simulink model "Q1_part2"  (R2022b)
settings: Solver=VariableStepAuto  StartTime=0.0  StopTime=50  RelTol=1e-3
libraries: mpclib x11, simulink x6, slpidlib x4
settings Model: Creator=Alireza  LastModifiedBy=Alireza

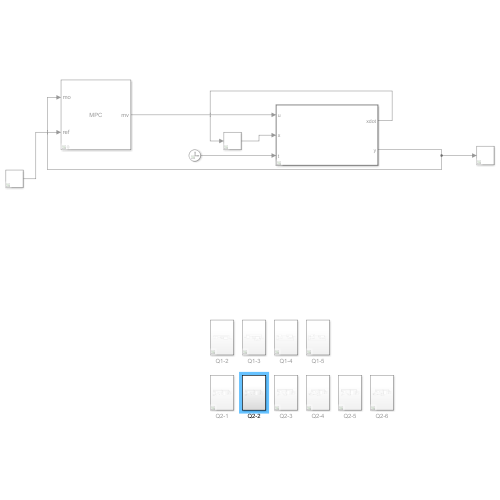
[thumbnail: Simulink's stored preview of the top-level diagram]
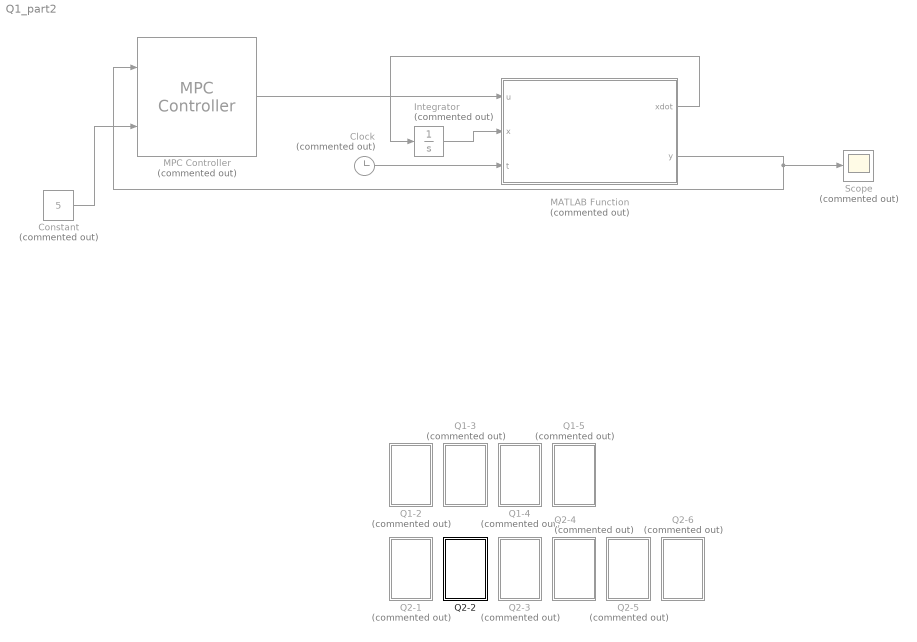
== system Q1_part2 ==
  Clock : Clock  Commented=on
  Constant : Constant  Commented=on  Value=5
  Integrator : Integrator  Commented=on  InitialCondition=[0 0 0 0]
  MATLAB Function : MATLAB Function  Commented=on  TreatAsAtomicUnit=on
  MPC Controller : mpclib/MPC Controller  Commented=on  SCDEnableBlockLinearizationSpecification=on  is_multiple=0  enable_value=0  return_u0=off  updateMPCinCallerWorkspace=on  md_inport=off  mv_inport=off  uref_inport=off  return_cost=off  return_mvseq=off  return_qpstatus=off  return_xseq=off  return_state=off  return_ovseq=off  state_inport=off  umin_inport=off  umax_inport=off  ymin_inport=off  ymax_inport=off  cc_inport=off  ywt_inport=off  uwt_inport=off  duwt_inport=off  rhoeps_inport=off  pm_inport=off  MaximumP=10  HorizonChoice=FixedHorizon  n_ts=0.01  n_p=100  n_mv=1  n_md=1  n_ud=0  n_mo=1  n_uo=0  BlockDataType=double  SampleTimeInherited=off  switch_inport=off
  Q1-2 : Subsystem  Commented=on
  Q1-3 : Subsystem  Commented=on
  Q1-4 : Subsystem  Commented=on
  Q1-5 : Subsystem  Commented=on
  Q2-1 : Subsystem  Commented=on
  Q2-2 : Subsystem
  Q2-3 : Subsystem  Commented=on
  Q2-4 : Subsystem  Commented=on
  Q2-5 : Subsystem  Commented=on
  Q2-6 : Subsystem  Commented=on
  Scope : Scope  Commented=on
  wires:
  Clock/1 -> MATLAB Function/3(t)
  Integrator/1 -> MATLAB Function/2(x)
  MATLAB Function/1(xdot) -> Integrator/1
  MATLAB Function/2(y) -> Scope/1, MPC Controller/1
  Constant/1 -> MPC Controller/2
  MPC Controller/1 -> MATLAB Function/1(u)

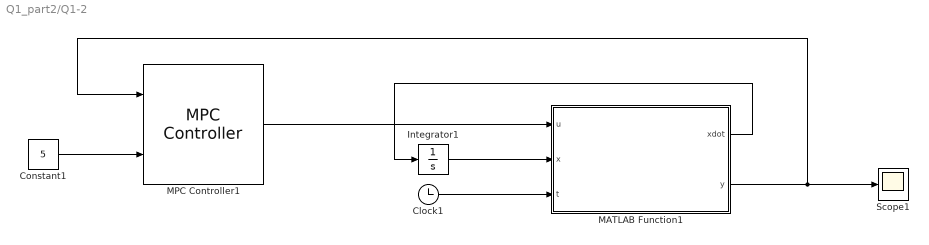
== system Q1_part2/Q1-2 ==
  Clock1 : Clock
  Constant1 : Constant  Value=5
  Integrator1 : Integrator  InitialCondition=[0 0 0 0]
  MATLAB Function1 : MATLAB Function  TreatAsAtomicUnit=on
  MPC Controller1 : mpclib/MPC Controller  SCDEnableBlockLinearizationSpecification=on  mpcobj=mpc1  is_multiple=0  enable_value=0  return_u0=off  updateMPCinCallerWorkspace=on  md_inport=off  mv_inport=off  uref_inport=off  return_cost=off  return_mvseq=off  return_qpstatus=off  return_xseq=off  return_state=off  return_ovseq=off  state_inport=off  umin_inport=off  umax_inport=off  ymin_inport=off  ymax_inport=off  cc_inport=off  ywt_inport=off  uwt_inport=off  duwt_inport=off  rhoeps_inport=off  pm_inport=off  MaximumP=10  HorizonChoice=FixedHorizon  n_ts=0.01  n_p=200  n_mv=1  n_md=0  n_ud=0  n_mo=1  n_uo=0  BlockDataType=double  SampleTimeInherited=off  switch_inport=off
  Scope1 : Scope
  wires:
  Clock1/1 -> MATLAB Function1/3(t)
  MATLAB Function1/2(y) -> MPC Controller1/1, Scope1/1
  Constant1/1 -> MPC Controller1/2
  Integrator1/1 -> MATLAB Function1/2(x)
  MPC Controller1/1 -> MATLAB Function1/1(u)
  MATLAB Function1/1(xdot) -> Integrator1/1

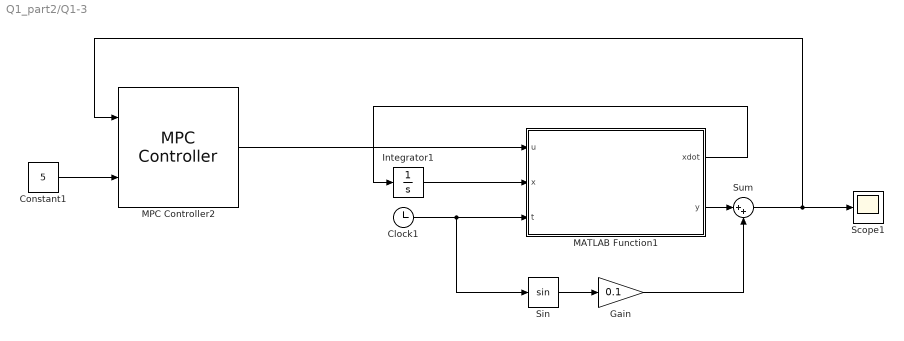
== system Q1_part2/Q1-3 ==
  Clock1 : Clock
  Constant1 : Constant  Value=5
  Gain : Gain  Gain=0.1
  Integrator1 : Integrator  InitialCondition=[0 0 0 0]
  MATLAB Function1 : MATLAB Function  TreatAsAtomicUnit=on
  MPC Controller2 : mpclib/MPC Controller  SCDEnableBlockLinearizationSpecification=on  mpcobj=mpc1  is_multiple=0  enable_value=0  return_u0=off  updateMPCinCallerWorkspace=on  md_inport=off  mv_inport=off  uref_inport=off  return_cost=off  return_mvseq=off  return_qpstatus=off  return_xseq=off  return_state=off  return_ovseq=off  state_inport=off  umin_inport=off  umax_inport=off  ymin_inport=off  ymax_inport=off  cc_inport=off  ywt_inport=off  uwt_inport=off  duwt_inport=off  rhoeps_inport=off  pm_inport=off  MaximumP=10  HorizonChoice=FixedHorizon  n_ts=0.01  n_p=200  n_mv=1  n_md=0  n_ud=0  n_mo=1  n_uo=0  BlockDataType=double  SampleTimeInherited=off  switch_inport=off
  Scope1 : Scope
  Sin : Trigonometry
  Sum : Sum  Inputs=|++
  wires:
  Clock1/1 -> Sin/1, MATLAB Function1/3(t)
  Constant1/1 -> MPC Controller2/2
  Integrator1/1 -> MATLAB Function1/2(x)
  MPC Controller2/1 -> MATLAB Function1/1(u)
  MATLAB Function1/1(xdot) -> Integrator1/1
  Sin/1 -> Gain/1
  Gain/1 -> Sum/2
  MATLAB Function1/2(y) -> Sum/1
  Sum/1 -> MPC Controller2/1, Scope1/1

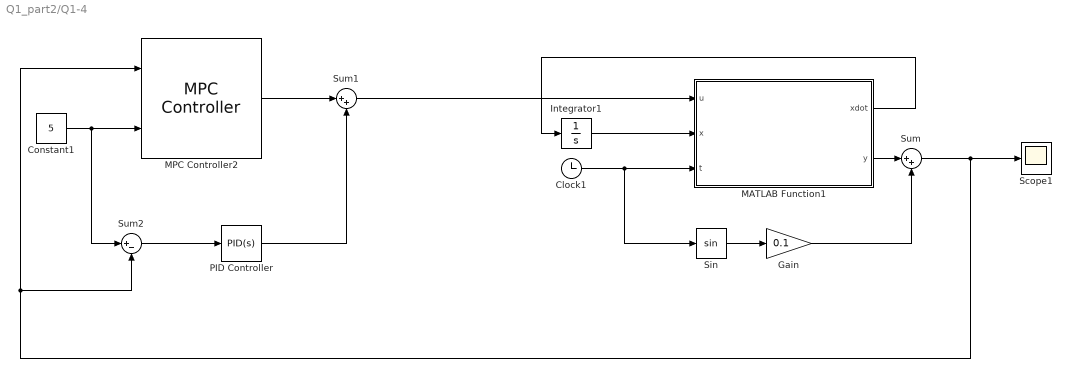
== system Q1_part2/Q1-4 ==
  Clock1 : Clock
  Constant1 : Constant  Value=5
  Gain : Gain  Gain=0.1
  Integrator1 : Integrator  InitialCondition=[0 0 0 0]
  MATLAB Function1 : MATLAB Function  TreatAsAtomicUnit=on
  MPC Controller2 : mpclib/MPC Controller  SCDEnableBlockLinearizationSpecification=on  mpcobj=mpc1  is_multiple=0  enable_value=0  return_u0=off  updateMPCinCallerWorkspace=on  md_inport=off  mv_inport=off  uref_inport=off  return_cost=off  return_mvseq=off  return_qpstatus=off  return_xseq=off  return_state=off  return_ovseq=off  state_inport=off  umin_inport=off  umax_inport=off  ymin_inport=off  ymax_inport=off  cc_inport=off  ywt_inport=off  uwt_inport=off  duwt_inport=off  rhoeps_inport=off  pm_inport=off  MaximumP=10  HorizonChoice=FixedHorizon  n_ts=0.01  n_p=200  n_mv=1  n_md=0  n_ud=0  n_mo=1  n_uo=0  BlockDataType=double  SampleTimeInherited=off  switch_inport=off
  PID Controller : slpidlib/PID Controller  Controller=PID  Form=Parallel  TimeDomain=Continuous-time  UseExternalTs=off  SampleTime=-1  IntegratorMethod=Forward Euler  FilterMethod=Forward Euler  ControllerParametersSource=internal  P=14.0581841806132  I=1.12903294333541  UseKiTs=off  D=19.0426786123122  N=1197.69951514709  UseFilter=on  TunerSelectOption=Transfer Function Based (PID Tuner App)  InitialConditionSource=internal  InitialConditionForIntegrator=0  InitialConditionForFilter=0  DifferentiatorICPrevScaledInput=0  ExternalReset=none  TrackingMode=off  Kt=1  LimitOutput=off  SatLimitsSource=internal  UpperSaturationLimit=inf  LowerSaturationLimit=-inf  LinearizeAsGain=on  AntiWindupMode=none  Kb=1  LimitIntegrator=off  UpperIntegratorSaturationLimit=inf  LowerIntegratorSaturationLimit=-inf  POutMin=[]  POutMax=[]  IOutMin=[]  IOutMax=[]  DOutMin=[]  DOutMax=[]  NOutMin=[]  NOutMax=[]  SumOutMin=[]  SumOutMax=[]  SaturationOutMin=[]  SaturationOutMax=[]  PParamMin=[]  PParamMax=[]  IParamMin=[]  IParamMax=[]  DParamMin=[]  DParamMax=[]  NParamMin=[]  NParamMax=[]  KbParamMin=[]  KbParamMax=[]  KtParamMin=[]  KtParamMax=[]  KbOutMin=[]  KbOutMax=[]  KtOutMin=[]  KtOutMax=[]  IntegratorOutMin=[]  IntegratorOutMax=[]  FilterOutMin=[]  FilterOutMax=[]  SumI1OutMin=[]  SumI1OutMax=[]  SumI2OutMin=[]  SumI2OutMax=[]  SumI3OutMin=[]  SumI3OutMax=[]  SumI4OutMin=[]  SumI4OutMax=[]  SumDOutMin=[]  SumDOutMax=[]  DifferentiatorOutMin=[]  DifferentiatorOutMax=[]  FilterDiffOutCoefMin=[]  FilterDiffOutCoefMax=[]  ReciprocalOutMin=[]  ReciprocalOutMax=[]  SumDenOutMin=[]  SumDenOutMax=[]  SumNumOutMin=[]  SumNumOutMax=[]  DivideOutMin=[]  DivideOutMax=[]  UdiffTsProdOutMin=[]  UdiffTsProdOutMax=[]  NTsProdOutMin=[]  NTsProdOutMax=[]  UintegralTsProdOutMin=[]  UintegralTsProdOutMax=[]  UngainTsProdOutMin=[]  UngainTsProdOutMax=[]  ClampingZeroOutDataTypeStr=Inherit: Inherit via back propagation  ClampingZeroOutMin=[]  ClampingZeroOutMax=[]  FilterDenConstantOutDataTypeStr=Inherit: Inherit via back propagation  FilterDenConstantOutMin=[]  FilterDenConstantOutMax=[]  PCopyOutDataTypeStr=Inherit: Inherit via back propagation  PCopyOutMin=[]  PCopyOutMax=[]  NCopyOutDataTypeStr=Inherit: Inherit via back propagation  NCopyOutMin=[]  NCopyOutMax=[]  IntegratorContinuousStateAttributes=''  IntegratorStateMustResolveToSignalObject=off  IntegratorRTWStateStorageClass=Auto  FilterContinuousStateAttributes=''  FilterStateMustResolveToSignalObject=off  FilterRTWStateStorageClass=Auto  ParallelPVariant=InternalParameters  IdealPVariant=Disabled  IVariant=InternalParameters  DVariant=InternalParameters  IntegratorVariant=Continuous  SatVariant=Disabled  AWVariant=Passthrough  PCopyVariant=Disabled  TRVariant=Disabled  FdbkBlocksVariant=Forward  IdealPFdbkVariant=Disabled  SatFdbkVariant=Disabled  DerivativeFilterVariant=ContFilter  NVariant=InternalParameters  NCopyVariant=Disabled  FilterICVariant=InternalICsFilter  IntegratorICVariant=InternalICs  ExternalResetVariant=Disabled  TRSumVariant=Passthrough  SumFdbkVariant=Disabled  SumVariant=Sum_PID  TsampFilterVariant=InternalTs  TsampNgainVariant=Passthrough  TsampIntegralVariant=Passthrough  ExternalSaturationOutDataTypeStr=Inherit: Same as second input
  Scope1 : Scope
  Sin : Trigonometry
  Sum : Sum  Inputs=|++
  Sum1 : Sum  Inputs=|++
  Sum2 : Sum  Inputs=|+-
  wires:
  Sum/1 -> Scope1/1, MPC Controller2/1, Sum2/2
  MATLAB Function1/2(y) -> Sum/1
  Gain/1 -> Sum/2
  Sin/1 -> Gain/1
  MATLAB Function1/1(xdot) -> Integrator1/1
  Integrator1/1 -> MATLAB Function1/2(x)
  Constant1/1 -> Sum2/1, MPC Controller2/2
  Clock1/1 -> MATLAB Function1/3(t), Sin/1
  MPC Controller2/1 -> Sum1/1
  PID Controller/1 -> Sum1/2
  Sum1/1 -> MATLAB Function1/1(u)
  Sum2/1 -> PID Controller/1

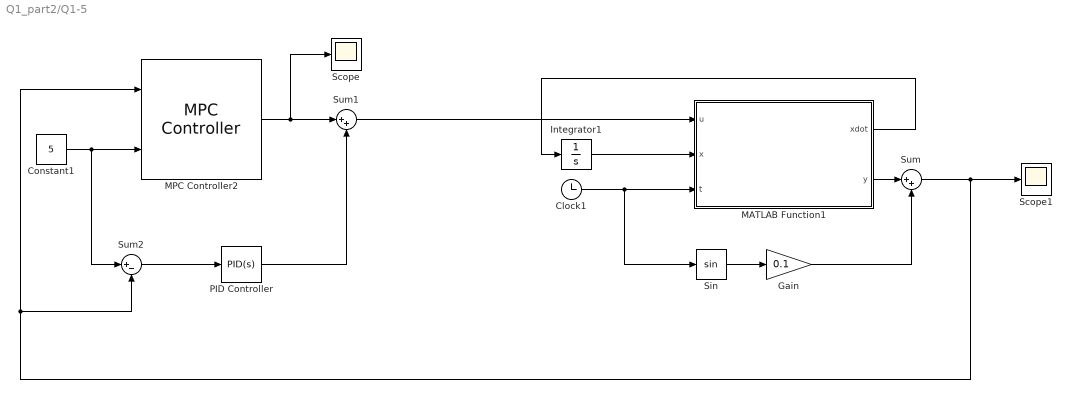
== system Q1_part2/Q1-5 ==
  Clock1 : Clock
  Constant1 : Constant  Value=5
  Gain : Gain  Gain=0.1
  Integrator1 : Integrator  InitialCondition=[0 0 0 0]
  MATLAB Function1 : MATLAB Function  TreatAsAtomicUnit=on
  MPC Controller2 : mpclib/MPC Controller  SCDEnableBlockLinearizationSpecification=on  mpcobj=mpc2  is_multiple=0  enable_value=0  return_u0=off  updateMPCinCallerWorkspace=on  md_inport=off  mv_inport=off  uref_inport=off  return_cost=off  return_mvseq=off  return_qpstatus=off  return_xseq=off  return_state=off  return_ovseq=off  state_inport=off  umin_inport=off  umax_inport=off  ymin_inport=off  ymax_inport=off  cc_inport=off  ywt_inport=off  uwt_inport=off  duwt_inport=off  rhoeps_inport=off  pm_inport=off  MaximumP=10  HorizonChoice=FixedHorizon  n_ts=0.01  n_p=200  n_mv=1  n_md=0  n_ud=0  n_mo=1  n_uo=0  BlockDataType=double  SampleTimeInherited=off  switch_inport=off
  PID Controller : slpidlib/PID Controller  Controller=PID  Form=Parallel  TimeDomain=Continuous-time  UseExternalTs=off  SampleTime=-1  IntegratorMethod=Forward Euler  FilterMethod=Forward Euler  ControllerParametersSource=internal  P=14.0581841806132  I=1.12903294333541  UseKiTs=off  D=19.0426786123122  N=1197.69951514709  UseFilter=on  TunerSelectOption=Transfer Function Based (PID Tuner App)  InitialConditionSource=internal  InitialConditionForIntegrator=0  InitialConditionForFilter=0  DifferentiatorICPrevScaledInput=0  ExternalReset=none  TrackingMode=off  Kt=1  LimitOutput=off  SatLimitsSource=internal  UpperSaturationLimit=inf  LowerSaturationLimit=-inf  LinearizeAsGain=on  AntiWindupMode=none  Kb=1  LimitIntegrator=off  UpperIntegratorSaturationLimit=inf  LowerIntegratorSaturationLimit=-inf  POutMin=[]  POutMax=[]  IOutMin=[]  IOutMax=[]  DOutMin=[]  DOutMax=[]  NOutMin=[]  NOutMax=[]  SumOutMin=[]  SumOutMax=[]  SaturationOutMin=[]  SaturationOutMax=[]  PParamMin=[]  PParamMax=[]  IParamMin=[]  IParamMax=[]  DParamMin=[]  DParamMax=[]  NParamMin=[]  NParamMax=[]  KbParamMin=[]  KbParamMax=[]  KtParamMin=[]  KtParamMax=[]  KbOutMin=[]  KbOutMax=[]  KtOutMin=[]  KtOutMax=[]  IntegratorOutMin=[]  IntegratorOutMax=[]  FilterOutMin=[]  FilterOutMax=[]  SumI1OutMin=[]  SumI1OutMax=[]  SumI2OutMin=[]  SumI2OutMax=[]  SumI3OutMin=[]  SumI3OutMax=[]  SumI4OutMin=[]  SumI4OutMax=[]  SumDOutMin=[]  SumDOutMax=[]  DifferentiatorOutMin=[]  DifferentiatorOutMax=[]  FilterDiffOutCoefMin=[]  FilterDiffOutCoefMax=[]  ReciprocalOutMin=[]  ReciprocalOutMax=[]  SumDenOutMin=[]  SumDenOutMax=[]  SumNumOutMin=[]  SumNumOutMax=[]  DivideOutMin=[]  DivideOutMax=[]  UdiffTsProdOutMin=[]  UdiffTsProdOutMax=[]  NTsProdOutMin=[]  NTsProdOutMax=[]  UintegralTsProdOutMin=[]  UintegralTsProdOutMax=[]  UngainTsProdOutMin=[]  UngainTsProdOutMax=[]  ClampingZeroOutDataTypeStr=Inherit: Inherit via back propagation  ClampingZeroOutMin=[]  ClampingZeroOutMax=[]  FilterDenConstantOutDataTypeStr=Inherit: Inherit via back propagation  FilterDenConstantOutMin=[]  FilterDenConstantOutMax=[]  PCopyOutDataTypeStr=Inherit: Inherit via back propagation  PCopyOutMin=[]  PCopyOutMax=[]  NCopyOutDataTypeStr=Inherit: Inherit via back propagation  NCopyOutMin=[]  NCopyOutMax=[]  IntegratorContinuousStateAttributes=''  IntegratorStateMustResolveToSignalObject=off  IntegratorRTWStateStorageClass=Auto  FilterContinuousStateAttributes=''  FilterStateMustResolveToSignalObject=off  FilterRTWStateStorageClass=Auto  ParallelPVariant=InternalParameters  IdealPVariant=Disabled  IVariant=InternalParameters  DVariant=InternalParameters  IntegratorVariant=Continuous  SatVariant=Disabled  AWVariant=Passthrough  PCopyVariant=Disabled  TRVariant=Disabled  FdbkBlocksVariant=Forward  IdealPFdbkVariant=Disabled  SatFdbkVariant=Disabled  DerivativeFilterVariant=ContFilter  NVariant=InternalParameters  NCopyVariant=Disabled  FilterICVariant=InternalICsFilter  IntegratorICVariant=InternalICs  ExternalResetVariant=Disabled  TRSumVariant=Passthrough  SumFdbkVariant=Disabled  SumVariant=Sum_PID  TsampFilterVariant=InternalTs  TsampNgainVariant=Passthrough  TsampIntegralVariant=Passthrough  ExternalSaturationOutDataTypeStr=Inherit: Same as second input
  Scope : Scope
  Scope1 : Scope
  Sin : Trigonometry
  Sum : Sum  Inputs=|++
  Sum1 : Sum  Inputs=|++
  Sum2 : Sum  Inputs=|+-
  wires:
  Sum2/1 -> PID Controller/1
  Sum1/1 -> MATLAB Function1/1(u)
  PID Controller/1 -> Sum1/2
  MPC Controller2/1 -> Scope/1, Sum1/1
  Clock1/1 -> Sin/1, MATLAB Function1/3(t)
  Constant1/1 -> MPC Controller2/2, Sum2/1
  Integrator1/1 -> MATLAB Function1/2(x)
  MATLAB Function1/1(xdot) -> Integrator1/1
  Sin/1 -> Gain/1
  Gain/1 -> Sum/2
  MATLAB Function1/2(y) -> Sum/1
  Sum/1 -> Sum2/2, MPC Controller2/1, Scope1/1

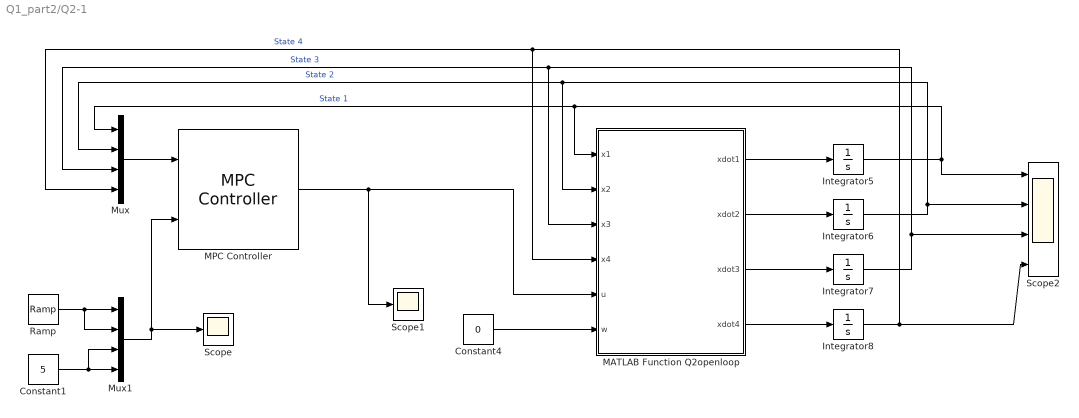
== system Q1_part2/Q2-1 ==
  Constant1 : Constant  Value=5
  Constant4 : Constant  Value=0
  Integrator{5..8} (4 alike) : Integrator
  MATLAB Function Q2openloop : MATLAB Function  TreatAsAtomicUnit=on
  MPC Controller : mpclib/MPC Controller  SCDEnableBlockLinearizationSpecification=on  mpcobj=mpc1  is_multiple=0  enable_value=0  return_u0=off  updateMPCinCallerWorkspace=on  md_inport=off  mv_inport=off  uref_inport=off  return_cost=off  return_mvseq=off  return_qpstatus=off  return_xseq=off  return_state=off  return_ovseq=off  state_inport=off  umin_inport=off  umax_inport=off  ymin_inport=off  ymax_inport=off  cc_inport=off  ywt_inport=off  uwt_inport=off  duwt_inport=off  rhoeps_inport=off  pm_inport=off  MaximumP=10  HorizonChoice=FixedHorizon  n_ts=0.01  n_p=650  n_mv=1  n_md=0  n_ud=0  n_mo=4  n_uo=0  BlockDataType=double  SampleTimeInherited=off  switch_inport=off
  Mux : Mux
  Mux1 : Mux
  Ramp : simulink/Sources/Ramp  slope=1  start=0  InitialOutput=0
  Scope : Scope
  Scope1 : Scope
  Scope2 : Scope  NumInputPorts=4
  wires:
  Mux/1 -> MPC Controller/1
  Ramp/1 -> Mux1/2, Mux1/1
  Constant1/1 -> Mux1/4, Mux1/3
  Mux1/1 -> Scope/1, MPC Controller/2
  Integrator5/1 -> Scope2/1, Mux/1, MATLAB Function Q2openloop/1(x1)  "State 1"
  MATLAB Function Q2openloop/1(xdot1) -> Integrator5/1
  Integrator7/1 -> Scope2/3, MATLAB Function Q2openloop/3(x3), Mux/3  "State 3"
  Integrator6/1 -> Scope2/2, MATLAB Function Q2openloop/2(x2), Mux/2  "State 2"
  MATLAB Function Q2openloop/3(xdot3) -> Integrator7/1
  MATLAB Function Q2openloop/4(xdot4) -> Integrator8/1
  MATLAB Function Q2openloop/2(xdot2) -> Integrator6/1
  Integrator8/1 -> MATLAB Function Q2openloop/4(x4), Mux/4, Scope2/4  "State 4"
  Constant4/1 -> MATLAB Function Q2openloop/6(w)
  MPC Controller/1 -> MATLAB Function Q2openloop/5(u), Scope1/1

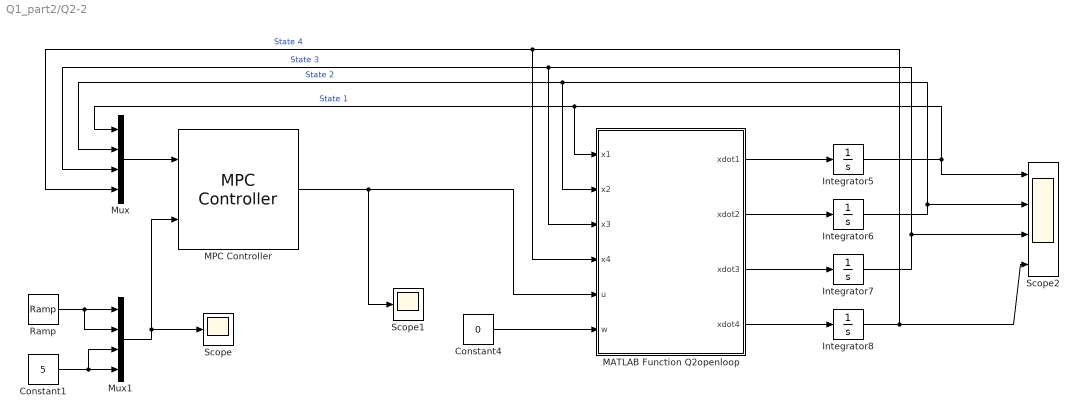
== system Q1_part2/Q2-2 ==
  Constant1 : Constant  Value=5
  Constant4 : Constant  Value=0
  Integrator{5..8} (4 alike) : Integrator
  MATLAB Function Q2openloop : MATLAB Function  TreatAsAtomicUnit=on
  MPC Controller : mpclib/MPC Controller  SCDEnableBlockLinearizationSpecification=on  mpcobj=mpc1  is_multiple=0  enable_value=0  return_u0=off  updateMPCinCallerWorkspace=on  md_inport=off  mv_inport=off  uref_inport=off  return_cost=off  return_mvseq=off  return_qpstatus=off  return_xseq=off  return_state=off  return_ovseq=off  state_inport=off  umin_inport=off  umax_inport=off  ymin_inport=off  ymax_inport=off  cc_inport=off  ywt_inport=off  uwt_inport=off  duwt_inport=off  rhoeps_inport=off  pm_inport=off  MaximumP=10  HorizonChoice=FixedHorizon  n_ts=0.01  n_p=650  n_mv=1  n_md=0  n_ud=0  n_mo=4  n_uo=0  BlockDataType=double  SampleTimeInherited=off  switch_inport=off
  Mux : Mux
  Mux1 : Mux
  Ramp : simulink/Sources/Ramp  slope=1  start=0  InitialOutput=0
  Scope : Scope
  Scope1 : Scope
  Scope2 : Scope  NumInputPorts=4
  wires:
  MPC Controller/1 -> Scope1/1, MATLAB Function Q2openloop/5(u)
  Constant4/1 -> MATLAB Function Q2openloop/6(w)
  Integrator8/1 -> Scope2/4, Mux/4, MATLAB Function Q2openloop/4(x4)  "State 4"
  MATLAB Function Q2openloop/2(xdot2) -> Integrator6/1
  MATLAB Function Q2openloop/4(xdot4) -> Integrator8/1
  MATLAB Function Q2openloop/3(xdot3) -> Integrator7/1
  Integrator6/1 -> Mux/2, MATLAB Function Q2openloop/2(x2), Scope2/2  "State 2"
  Integrator7/1 -> Mux/3, MATLAB Function Q2openloop/3(x3), Scope2/3  "State 3"
  MATLAB Function Q2openloop/1(xdot1) -> Integrator5/1
  Integrator5/1 -> MATLAB Function Q2openloop/1(x1), Mux/1, Scope2/1  "State 1"
  Mux1/1 -> MPC Controller/2, Scope/1
  Constant1/1 -> Mux1/3, Mux1/4
  Ramp/1 -> Mux1/1, Mux1/2
  Mux/1 -> MPC Controller/1

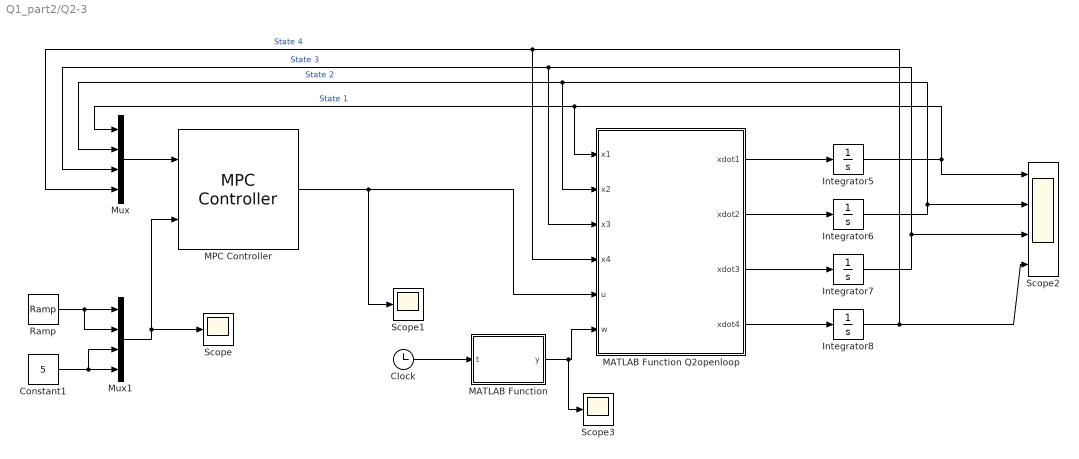
== system Q1_part2/Q2-3 ==
  Clock : Clock
  Constant1 : Constant  Value=5
  Integrator{5..8} (4 alike) : Integrator
  MATLAB Function : MATLAB Function  TreatAsAtomicUnit=on
  MATLAB Function Q2openloop : MATLAB Function  TreatAsAtomicUnit=on
  MPC Controller : mpclib/MPC Controller  SCDEnableBlockLinearizationSpecification=on  mpcobj=mpc1  is_multiple=0  enable_value=0  return_u0=off  updateMPCinCallerWorkspace=on  md_inport=off  mv_inport=off  uref_inport=off  return_cost=off  return_mvseq=off  return_qpstatus=off  return_xseq=off  return_state=off  return_ovseq=off  state_inport=off  umin_inport=off  umax_inport=off  ymin_inport=off  ymax_inport=off  cc_inport=off  ywt_inport=off  uwt_inport=off  duwt_inport=off  rhoeps_inport=off  pm_inport=off  MaximumP=10  HorizonChoice=FixedHorizon  n_ts=0.01  n_p=650  n_mv=1  n_md=0  n_ud=0  n_mo=4  n_uo=0  BlockDataType=double  SampleTimeInherited=off  switch_inport=off
  Mux : Mux
  Mux1 : Mux
  Ramp : simulink/Sources/Ramp  slope=1  start=0  InitialOutput=0
  Scope : Scope
  Scope1 : Scope
  Scope2 : Scope  NumInputPorts=4
  Scope3 : Scope
  wires:
  Mux/1 -> MPC Controller/1
  Ramp/1 -> Mux1/2, Mux1/1
  Constant1/1 -> Mux1/4, Mux1/3
  Mux1/1 -> Scope/1, MPC Controller/2
  Integrator5/1 -> Scope2/1, Mux/1, MATLAB Function Q2openloop/1(x1)  "State 1"
  MATLAB Function Q2openloop/1(xdot1) -> Integrator5/1
  Integrator7/1 -> Scope2/3, MATLAB Function Q2openloop/3(x3), Mux/3  "State 3"
  Integrator6/1 -> Scope2/2, MATLAB Function Q2openloop/2(x2), Mux/2  "State 2"
  MATLAB Function Q2openloop/3(xdot3) -> Integrator7/1
  MATLAB Function Q2openloop/4(xdot4) -> Integrator8/1
  MATLAB Function Q2openloop/2(xdot2) -> Integrator6/1
  Integrator8/1 -> MATLAB Function Q2openloop/4(x4), Mux/4, Scope2/4  "State 4"
  MPC Controller/1 -> MATLAB Function Q2openloop/5(u), Scope1/1
  MATLAB Function/1(y) -> Scope3/1, MATLAB Function Q2openloop/6(w)
  Clock/1 -> MATLAB Function/1(t)

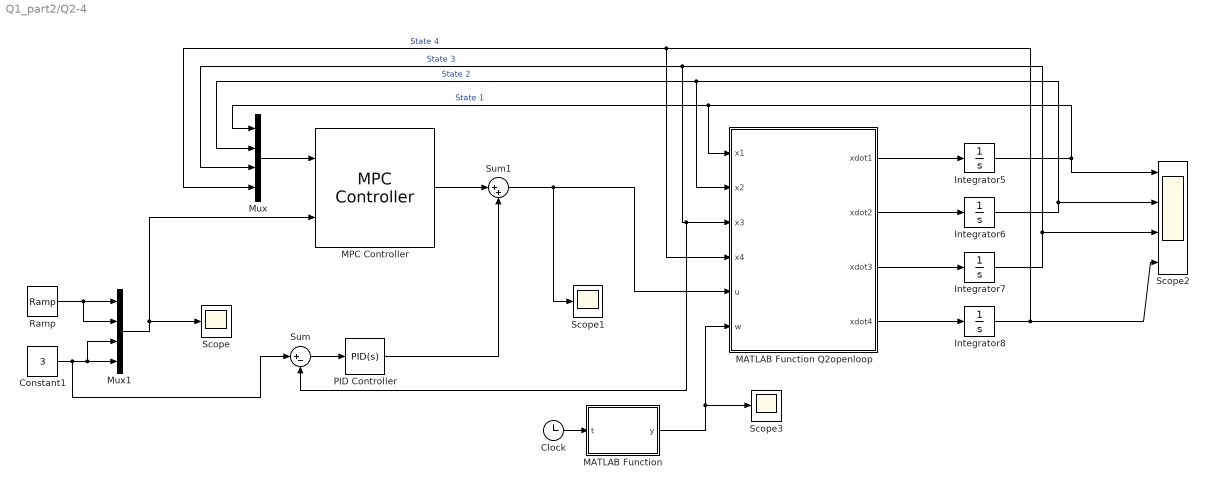
== system Q1_part2/Q2-4 ==
  Clock : Clock
  Constant1 : Constant  Value=3
  Integrator{5..8} (4 alike) : Integrator
  MATLAB Function : MATLAB Function  TreatAsAtomicUnit=on
  MATLAB Function Q2openloop : MATLAB Function  TreatAsAtomicUnit=on
  MPC Controller : mpclib/MPC Controller  SCDEnableBlockLinearizationSpecification=on  mpcobj=mpc1  is_multiple=0  enable_value=0  return_u0=off  updateMPCinCallerWorkspace=on  md_inport=off  mv_inport=off  uref_inport=off  return_cost=off  return_mvseq=off  return_qpstatus=off  return_xseq=off  return_state=off  return_ovseq=off  state_inport=off  umin_inport=off  umax_inport=off  ymin_inport=off  ymax_inport=off  cc_inport=off  ywt_inport=off  uwt_inport=off  duwt_inport=off  rhoeps_inport=off  pm_inport=off  MaximumP=10  HorizonChoice=FixedHorizon  n_ts=0.01  n_p=650  n_mv=1  n_md=0  n_ud=0  n_mo=4  n_uo=0  BlockDataType=double  SampleTimeInherited=off  switch_inport=off
  Mux : Mux
  Mux1 : Mux
  PID Controller : slpidlib/PID Controller  Controller=PID  Form=Parallel  TimeDomain=Continuous-time  UseExternalTs=off  SampleTime=-1  IntegratorMethod=Forward Euler  FilterMethod=Forward Euler  ControllerParametersSource=internal  P=200  I=10  UseKiTs=off  D=100  N=100  UseFilter=on  TunerSelectOption=Transfer Function Based (PID Tuner App)  InitialConditionSource=internal  InitialConditionForIntegrator=0  InitialConditionForFilter=0  DifferentiatorICPrevScaledInput=0  ExternalReset=none  TrackingMode=off  Kt=1  LimitOutput=off  SatLimitsSource=internal  UpperSaturationLimit=inf  LowerSaturationLimit=-inf  LinearizeAsGain=on  AntiWindupMode=none  Kb=1  LimitIntegrator=off  UpperIntegratorSaturationLimit=inf  LowerIntegratorSaturationLimit=-inf  POutMin=[]  POutMax=[]  IOutMin=[]  IOutMax=[]  DOutMin=[]  DOutMax=[]  NOutMin=[]  NOutMax=[]  SumOutMin=[]  SumOutMax=[]  SaturationOutMin=[]  SaturationOutMax=[]  PParamMin=[]  PParamMax=[]  IParamMin=[]  IParamMax=[]  DParamMin=[]  DParamMax=[]  NParamMin=[]  NParamMax=[]  KbParamMin=[]  KbParamMax=[]  KtParamMin=[]  KtParamMax=[]  KbOutMin=[]  KbOutMax=[]  KtOutMin=[]  KtOutMax=[]  IntegratorOutMin=[]  IntegratorOutMax=[]  FilterOutMin=[]  FilterOutMax=[]  SumI1OutMin=[]  SumI1OutMax=[]  SumI2OutMin=[]  SumI2OutMax=[]  SumI3OutMin=[]  SumI3OutMax=[]  SumI4OutMin=[]  SumI4OutMax=[]  SumDOutMin=[]  SumDOutMax=[]  DifferentiatorOutMin=[]  DifferentiatorOutMax=[]  FilterDiffOutCoefMin=[]  FilterDiffOutCoefMax=[]  ReciprocalOutMin=[]  ReciprocalOutMax=[]  SumDenOutMin=[]  SumDenOutMax=[]  SumNumOutMin=[]  SumNumOutMax=[]  DivideOutMin=[]  DivideOutMax=[]  UdiffTsProdOutMin=[]  UdiffTsProdOutMax=[]  NTsProdOutMin=[]  NTsProdOutMax=[]  UintegralTsProdOutMin=[]  UintegralTsProdOutMax=[]  UngainTsProdOutMin=[]  UngainTsProdOutMax=[]  ClampingZeroOutDataTypeStr=Inherit: Inherit via back propagation  ClampingZeroOutMin=[]  ClampingZeroOutMax=[]  FilterDenConstantOutDataTypeStr=Inherit: Inherit via back propagation  FilterDenConstantOutMin=[]  FilterDenConstantOutMax=[]  PCopyOutDataTypeStr=Inherit: Inherit via back propagation  PCopyOutMin=[]  PCopyOutMax=[]  NCopyOutDataTypeStr=Inherit: Inherit via back propagation  NCopyOutMin=[]  NCopyOutMax=[]  IntegratorContinuousStateAttributes=''  IntegratorStateMustResolveToSignalObject=off  IntegratorRTWStateStorageClass=Auto  FilterContinuousStateAttributes=''  FilterStateMustResolveToSignalObject=off  FilterRTWStateStorageClass=Auto  ParallelPVariant=InternalParameters  IdealPVariant=Disabled  IVariant=InternalParameters  DVariant=InternalParameters  IntegratorVariant=Continuous  SatVariant=Disabled  AWVariant=Passthrough  PCopyVariant=Disabled  TRVariant=Disabled  FdbkBlocksVariant=Forward  IdealPFdbkVariant=Disabled  SatFdbkVariant=Disabled  DerivativeFilterVariant=ContFilter  NVariant=InternalParameters  NCopyVariant=Disabled  FilterICVariant=InternalICsFilter  IntegratorICVariant=InternalICs  ExternalResetVariant=Disabled  TRSumVariant=Passthrough  SumFdbkVariant=Disabled  SumVariant=Sum_PID  TsampFilterVariant=InternalTs  TsampNgainVariant=Passthrough  TsampIntegralVariant=Passthrough  ExternalSaturationOutDataTypeStr=Inherit: Same as second input
  Ramp : simulink/Sources/Ramp  slope=1  start=0  InitialOutput=0
  Scope : Scope
  Scope1 : Scope
  Scope2 : Scope  NumInputPorts=4
  Scope3 : Scope
  Sum : Sum  Inputs=|+-
  Sum1 : Sum  Inputs=|++
  wires:
  Clock/1 -> MATLAB Function/1(t)
  MATLAB Function/1(y) -> Scope3/1, MATLAB Function Q2openloop/6(w)
  Integrator8/1 -> Scope2/4, Mux/4, MATLAB Function Q2openloop/4(x4)  "State 4"
  MATLAB Function Q2openloop/2(xdot2) -> Integrator6/1
  MATLAB Function Q2openloop/4(xdot4) -> Integrator8/1
  MATLAB Function Q2openloop/3(xdot3) -> Integrator7/1
  Integrator6/1 -> Mux/2, MATLAB Function Q2openloop/2(x2), Scope2/2  "State 2"
  Integrator7/1 -> Mux/3, MATLAB Function Q2openloop/3(x3), Sum/2, Scope2/3  "State 3"
  MATLAB Function Q2openloop/1(xdot1) -> Integrator5/1
  Integrator5/1 -> MATLAB Function Q2openloop/1(x1), Mux/1, Scope2/1  "State 1"
  Mux1/1 -> MPC Controller/2, Scope/1
  Constant1/1 -> Sum/1, Mux1/3, Mux1/4
  Ramp/1 -> Mux1/1, Mux1/2
  Mux/1 -> MPC Controller/1
  Sum/1 -> PID Controller/1
  MPC Controller/1 -> Sum1/1
  Sum1/1 -> Scope1/1, MATLAB Function Q2openloop/5(u)
  PID Controller/1 -> Sum1/2

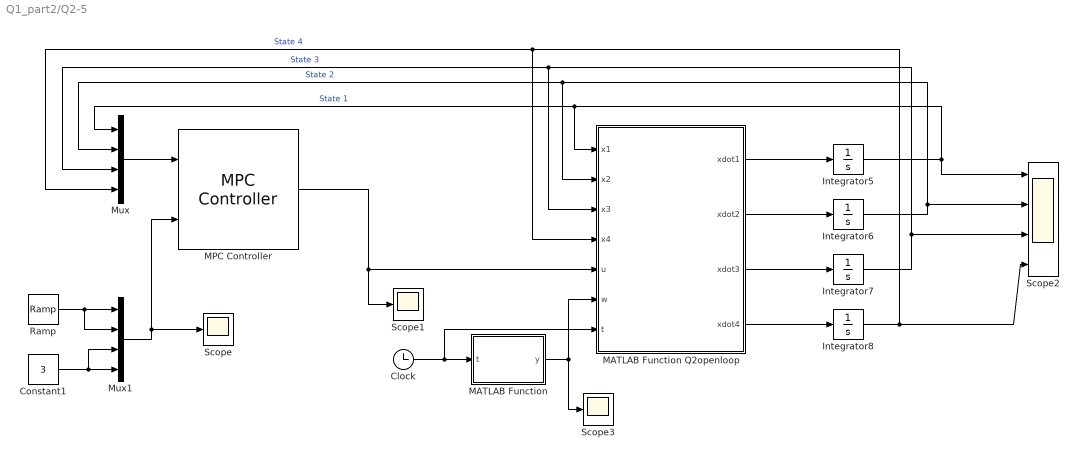
== system Q1_part2/Q2-5 ==
  Clock : Clock
  Constant1 : Constant  Value=3
  Integrator{5..8} (4 alike) : Integrator
  MATLAB Function : MATLAB Function  TreatAsAtomicUnit=on
  MATLAB Function Q2openloop : MATLAB Function  TreatAsAtomicUnit=on
  MPC Controller : mpclib/MPC Controller  SCDEnableBlockLinearizationSpecification=on  mpcobj=mpc1  is_multiple=0  enable_value=0  return_u0=off  updateMPCinCallerWorkspace=on  md_inport=off  mv_inport=off  uref_inport=off  return_cost=off  return_mvseq=off  return_qpstatus=off  return_xseq=off  return_state=off  return_ovseq=off  state_inport=off  umin_inport=off  umax_inport=off  ymin_inport=off  ymax_inport=off  cc_inport=off  ywt_inport=off  uwt_inport=off  duwt_inport=off  rhoeps_inport=off  pm_inport=off  MaximumP=10  HorizonChoice=FixedHorizon  n_ts=0.01  n_p=650  n_mv=1  n_md=0  n_ud=0  n_mo=4  n_uo=0  BlockDataType=double  SampleTimeInherited=off  switch_inport=off
  Mux : Mux
  Mux1 : Mux
  Ramp : simulink/Sources/Ramp  slope=1  start=0  InitialOutput=0
  Scope : Scope
  Scope1 : Scope
  Scope2 : Scope  NumInputPorts=4
  Scope3 : Scope
  wires:
  Clock/1 -> MATLAB Function Q2openloop/7(t), MATLAB Function/1(t)
  MATLAB Function/1(y) -> MATLAB Function Q2openloop/6(w), Scope3/1
  MPC Controller/1 -> Scope1/1, MATLAB Function Q2openloop/5(u)
  Integrator8/1 -> Scope2/4, Mux/4, MATLAB Function Q2openloop/4(x4)  "State 4"
  MATLAB Function Q2openloop/2(xdot2) -> Integrator6/1
  MATLAB Function Q2openloop/4(xdot4) -> Integrator8/1
  MATLAB Function Q2openloop/3(xdot3) -> Integrator7/1
  Integrator6/1 -> Mux/2, MATLAB Function Q2openloop/2(x2), Scope2/2  "State 2"
  Integrator7/1 -> Mux/3, MATLAB Function Q2openloop/3(x3), Scope2/3  "State 3"
  MATLAB Function Q2openloop/1(xdot1) -> Integrator5/1
  Integrator5/1 -> MATLAB Function Q2openloop/1(x1), Mux/1, Scope2/1  "State 1"
  Mux1/1 -> MPC Controller/2, Scope/1
  Constant1/1 -> Mux1/3, Mux1/4
  Ramp/1 -> Mux1/1, Mux1/2
  Mux/1 -> MPC Controller/1

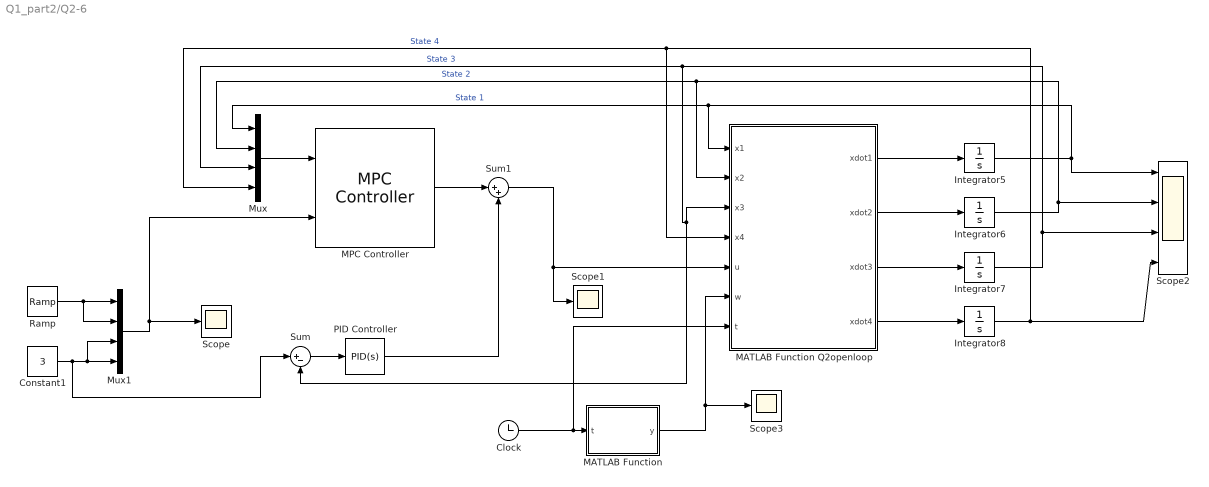
== system Q1_part2/Q2-6 ==
  Clock : Clock
  Constant1 : Constant  Value=3
  Integrator{5..8} (4 alike) : Integrator
  MATLAB Function : MATLAB Function  TreatAsAtomicUnit=on
  MATLAB Function Q2openloop : MATLAB Function  TreatAsAtomicUnit=on
  MPC Controller : mpclib/MPC Controller  SCDEnableBlockLinearizationSpecification=on  mpcobj=mpc1  is_multiple=0  enable_value=0  return_u0=off  updateMPCinCallerWorkspace=on  md_inport=off  mv_inport=off  uref_inport=off  return_cost=off  return_mvseq=off  return_qpstatus=off  return_xseq=off  return_state=off  return_ovseq=off  state_inport=off  umin_inport=off  umax_inport=off  ymin_inport=off  ymax_inport=off  cc_inport=off  ywt_inport=off  uwt_inport=off  duwt_inport=off  rhoeps_inport=off  pm_inport=off  MaximumP=10  HorizonChoice=FixedHorizon  n_ts=0.01  n_p=650  n_mv=1  n_md=0  n_ud=0  n_mo=4  n_uo=0  BlockDataType=double  SampleTimeInherited=off  switch_inport=off
  Mux : Mux
  Mux1 : Mux
  PID Controller : slpidlib/PID Controller  Controller=PID  Form=Parallel  TimeDomain=Continuous-time  UseExternalTs=off  SampleTime=-1  IntegratorMethod=Forward Euler  FilterMethod=Forward Euler  ControllerParametersSource=internal  P=200  I=10  UseKiTs=off  D=100  N=100  UseFilter=on  TunerSelectOption=Transfer Function Based (PID Tuner App)  InitialConditionSource=internal  InitialConditionForIntegrator=0  InitialConditionForFilter=0  DifferentiatorICPrevScaledInput=0  ExternalReset=none  TrackingMode=off  Kt=1  LimitOutput=off  SatLimitsSource=internal  UpperSaturationLimit=inf  LowerSaturationLimit=-inf  LinearizeAsGain=on  AntiWindupMode=none  Kb=1  LimitIntegrator=off  UpperIntegratorSaturationLimit=inf  LowerIntegratorSaturationLimit=-inf  POutMin=[]  POutMax=[]  IOutMin=[]  IOutMax=[]  DOutMin=[]  DOutMax=[]  NOutMin=[]  NOutMax=[]  SumOutMin=[]  SumOutMax=[]  SaturationOutMin=[]  SaturationOutMax=[]  PParamMin=[]  PParamMax=[]  IParamMin=[]  IParamMax=[]  DParamMin=[]  DParamMax=[]  NParamMin=[]  NParamMax=[]  KbParamMin=[]  KbParamMax=[]  KtParamMin=[]  KtParamMax=[]  KbOutMin=[]  KbOutMax=[]  KtOutMin=[]  KtOutMax=[]  IntegratorOutMin=[]  IntegratorOutMax=[]  FilterOutMin=[]  FilterOutMax=[]  SumI1OutMin=[]  SumI1OutMax=[]  SumI2OutMin=[]  SumI2OutMax=[]  SumI3OutMin=[]  SumI3OutMax=[]  SumI4OutMin=[]  SumI4OutMax=[]  SumDOutMin=[]  SumDOutMax=[]  DifferentiatorOutMin=[]  DifferentiatorOutMax=[]  FilterDiffOutCoefMin=[]  FilterDiffOutCoefMax=[]  ReciprocalOutMin=[]  ReciprocalOutMax=[]  SumDenOutMin=[]  SumDenOutMax=[]  SumNumOutMin=[]  SumNumOutMax=[]  DivideOutMin=[]  DivideOutMax=[]  UdiffTsProdOutMin=[]  UdiffTsProdOutMax=[]  NTsProdOutMin=[]  NTsProdOutMax=[]  UintegralTsProdOutMin=[]  UintegralTsProdOutMax=[]  UngainTsProdOutMin=[]  UngainTsProdOutMax=[]  ClampingZeroOutDataTypeStr=Inherit: Inherit via back propagation  ClampingZeroOutMin=[]  ClampingZeroOutMax=[]  FilterDenConstantOutDataTypeStr=Inherit: Inherit via back propagation  FilterDenConstantOutMin=[]  FilterDenConstantOutMax=[]  PCopyOutDataTypeStr=Inherit: Inherit via back propagation  PCopyOutMin=[]  PCopyOutMax=[]  NCopyOutDataTypeStr=Inherit: Inherit via back propagation  NCopyOutMin=[]  NCopyOutMax=[]  IntegratorContinuousStateAttributes=''  IntegratorStateMustResolveToSignalObject=off  IntegratorRTWStateStorageClass=Auto  FilterContinuousStateAttributes=''  FilterStateMustResolveToSignalObject=off  FilterRTWStateStorageClass=Auto  ParallelPVariant=InternalParameters  IdealPVariant=Disabled  IVariant=InternalParameters  DVariant=InternalParameters  IntegratorVariant=Continuous  SatVariant=Disabled  AWVariant=Passthrough  PCopyVariant=Disabled  TRVariant=Disabled  FdbkBlocksVariant=Forward  IdealPFdbkVariant=Disabled  SatFdbkVariant=Disabled  DerivativeFilterVariant=ContFilter  NVariant=InternalParameters  NCopyVariant=Disabled  FilterICVariant=InternalICsFilter  IntegratorICVariant=InternalICs  ExternalResetVariant=Disabled  TRSumVariant=Passthrough  SumFdbkVariant=Disabled  SumVariant=Sum_PID  TsampFilterVariant=InternalTs  TsampNgainVariant=Passthrough  TsampIntegralVariant=Passthrough  ExternalSaturationOutDataTypeStr=Inherit: Same as second input
  Ramp : simulink/Sources/Ramp  slope=1  start=0  InitialOutput=0
  Scope : Scope
  Scope1 : Scope
  Scope2 : Scope  NumInputPorts=4
  Scope3 : Scope
  Sum : Sum  Inputs=|+-
  Sum1 : Sum  Inputs=|++
  wires:
  PID Controller/1 -> Sum1/2
  Sum1/1 -> Scope1/1, MATLAB Function Q2openloop/5(u)
  MPC Controller/1 -> Sum1/1
  Sum/1 -> PID Controller/1
  Mux/1 -> MPC Controller/1
  Ramp/1 -> Mux1/2, Mux1/1
  Constant1/1 -> Mux1/4, Mux1/3, Sum/1
  Mux1/1 -> Scope/1, MPC Controller/2
  Integrator5/1 -> Scope2/1, Mux/1, MATLAB Function Q2openloop/1(x1)  "State 1"
  MATLAB Function Q2openloop/1(xdot1) -> Integrator5/1
  Integrator7/1 -> Scope2/3, Sum/2, MATLAB Function Q2openloop/3(x3), Mux/3  "State 3"
  Integrator6/1 -> Scope2/2, MATLAB Function Q2openloop/2(x2), Mux/2  "State 2"
  MATLAB Function Q2openloop/3(xdot3) -> Integrator7/1
  MATLAB Function Q2openloop/4(xdot4) -> Integrator8/1
  MATLAB Function Q2openloop/2(xdot2) -> Integrator6/1
  Integrator8/1 -> MATLAB Function Q2openloop/4(x4), Mux/4, Scope2/4  "State 4"
  MATLAB Function/1(y) -> MATLAB Function Q2openloop/6(w), Scope3/1
  Clock/1 -> MATLAB Function Q2openloop/7(t), MATLAB Function/1(t)

== matlab function Q1_part2/Q2-3/MATLAB Function ==
  data: t input; y output
function y = fcn(t)

y =200* 2*sin(4*pi*t);

== matlab function Q1_part2/Q2-4/MATLAB Function ==
  data: t input; y output
function y = fcn(t)

y =200* 2*sin(4*pi*t);

== matlab function Q1_part2/Q2-4/MATLAB Function Q2openloop ==
  data: x1 input size=1; x2 input size=1; x3 input; x4 input; xdot1 output size=1; u input size=1; xdot2 output size=1; w input; xdot3 output; xdot4 output
function [xdot1, xdot2, xdot3, xdot4] = Q2_System_Model(x1, x2, x3, x4, u, w)

% Parameter Values

m1 = 10000;
m2 = 8000;
k = 500000;
c = 5000;

% State-Equations

xdot1 = x3;
xdot2 = x4;
xdot3 = (1 / m1) * (k * (-x1 + x2) + c * (-x3 + x4) + u + w);
xdot4 = (1 / m2) * (k * (x1 - x2) + c * (x3 - x4));

== matlab function Q1_part2/Q2-6/MATLAB Function ==
  data: t input; y output
function y = fcn(t)

y =200* 2*sin(4*pi*t);

== matlab function Q1_part2/Q2-6/MATLAB Function Q2openloop ==
  data: x1 input size=1; x2 input size=1; x3 input; x4 input; xdot1 output size=1; u input size=1; xdot2 output size=1; w input; xdot3 output; xdot4 output; t input
function [xdot1, xdot2, xdot3, xdot4] = fcn(x1, x2, x3, x4, u, w, t)

% Parameter Values with uncertainity

m1 = 10000;
m1 = m1 + (m1/10) * sin(t);
m2 = 8000;
m2 = m2 + (m2/10) * sin(t);
k = 500000;
k = k + (k/20) * sin(t);
c = 5000;
c = c + (c/20) * sin(t);

% State-Equations

xdot1 = x3;
xdot2 = x4;
xdot3 = (1 / m1) * (k * (-x1 + x2) + c * (-x3 + x4) + u + w);
xdot4 = (1 / m2) * (k * (x1 - x2) + c * (x3 - x4));

== matlab function Q1_part2/Q1-2/MATLAB Function1 ==
  data: xdot output size=4; u input size=1; y output size=1; x input size=4; t input size=1
function [xdot , y] = System_SS_Model(u, x, t)

% Parameter ranges pertaining to the linear transfer function

ke = 75 + 25 * sin(t);
Ks = 0.375 + 0.125 * sin(t);
Kp = 2.5*10^( -12) + 2.5*10^( -12) * sin(t);
C1 = 2*10^( -11) + 1*10^( -11) * sin(t);
d = 700 + 100 * sin(t);
ma = 20.0 + 0.1 * sin(t);
Ai = 0.00203 + 0.0001 * sin(t);
Ao = 0.00152 + 0.00008 * sin(t);
ksp = 0.0012 + 0.0001 * sin(t);
tau = 35 + 5 * sin(t);

% Definig the parameters calculated for the state - space equations
a1 = (tau * (Kp * ma + C1 * d) + (C1 * ma)) / (tau *C1 * ma);
a2 = (tau * (Kp * d + C1 * ke + Ai^2 + Ao^2) + (Kp *ma + C1 * d)) / (tau * C1 * ma);
a3 = (tau * Kp * ke + Kp * d + C1 * ke + Ai^2 + Ao^2) / (tau * C1 * ma);
a4 = (Kp * ke) / (tau * C1 * ma);
beta = (ksp * Ks * ke * (Ai + Ao)) / (tau * C1 * ma);

% State -Space Matrices

A = [
0,1,0,0;
0,0,1,0;
0,0,0,1;
-a4,-a3,-a2,-a1];

B = [0;0;0;beta];
C = [1,0,0,0];
% State -Space equations
xdot = A * x + B * u;
y = C *x;

== matlab function Q1_part2/Q2-5/MATLAB Function ==
  data: t input; y output
function y = fcn(t)

y =200* 2*sin(4*pi*t);

== matlab function Q1_part2/Q2-5/MATLAB Function Q2openloop ==
  data: x1 input size=1; x2 input size=1; x3 input; x4 input; xdot1 output size=1; u input size=1; xdot2 output size=1; w input; xdot3 output; xdot4 output; t input
function [xdot1, xdot2, xdot3, xdot4] = fcn(x1, x2, x3, x4, u, w, t)

% Parameter Values with uncertainity

m1 = 10000;
m1 = m1 + (m1/10) * sin(t);
m2 = 8000;
m2 = m2 + (m2/10) * sin(t);
k = 500000;
k = k + (k/20) * sin(t);
c = 5000;
c = c + (c/20) * sin(t);

% State-Equations

xdot1 = x3;
xdot2 = x4;
xdot3 = (1 / m1) * (k * (-x1 + x2) + c * (-x3 + x4) + u + w);
xdot4 = (1 / m2) * (k * (x1 - x2) + c * (x3 - x4));

== matlab function Q1_part2/MATLAB Function ==
  data: xdot output; u input; y output; x input; t input
function [xdot , y] = System_SS_Model(u, x, t)

% Parameter ranges pertaining to the linear transfer function

ke = 75 + 25 * sin(t);
Ks = 0.375 + 0.125 * sin(t);
Kp = 2.5*10^( -12) + 2.5*10^( -12) * sin(t);
C1 = 2*10^( -11) + 1*10^( -11) * sin(t);
d = 700 + 100 * sin(t);
ma = 20.0 + 0.1 * sin(t);
Ai = 0.00203 + 0.0001 * sin(t);
Ao = 0.00152 + 0.00008 * sin(t);
ksp = 0.0012 + 0.0001 * sin(t);
tau = 35 + 5 * sin(t);

% Definig the parameters calculated for the state - space equations
a1 = (tau * (Kp * ma + C1 * d) + (C1 * ma)) / (tau *C1 * ma);
a2 = (tau * (Kp * d + C1 * ke + Ai^2 + Ao^2) + (Kp *ma + C1 * d)) / (tau * C1 * ma);
a3 = (tau * Kp * ke + Kp * d + C1 * ke + Ai^2 + Ao^2) / (tau * C1 * ma);
a4 = (Kp * ke) / (tau * C1 * ma);
beta = (ksp * Ks * ke * (Ai + Ao)) / (tau * C1 * ma);

% State -Space Matrices

A = [
0,1,0,0;
0,0,1,0;
0,0,0,1;
-a4,-a3,-a2,-a1];

B = [0;0;0;beta];
C = [1,0,0,0];
% State -Space equations
xdot = A * x + B * u;
y = C *x;

== matlab function Q1_part2/Q1-3/MATLAB Function1 ==
  data: xdot output size=4; u input size=1; y output size=1; x input size=4; t input size=1
function [xdot , y] = System_SS_Model(u, x, t)

% Parameter ranges pertaining to the linear transfer function

ke = 75 + 25 * sin(t);
Ks = 0.375 + 0.125 * sin(t);
Kp = 2.5*10^( -12) + 2.5*10^( -12) * sin(t);
C1 = 2*10^( -11) + 1*10^( -11) * sin(t);
d = 700 + 100 * sin(t);
ma = 20.0 + 0.1 * sin(t);
Ai = 0.00203 + 0.0001 * sin(t);
Ao = 0.00152 + 0.00008 * sin(t);
ksp = 0.0012 + 0.0001 * sin(t);
tau = 35 + 5 * sin(t);

% Definig the parameters calculated for the state - space equations
a1 = (tau * (Kp * ma + C1 * d) + (C1 * ma)) / (tau *C1 * ma);
a2 = (tau * (Kp * d + C1 * ke + Ai^2 + Ao^2) + (Kp *ma + C1 * d)) / (tau * C1 * ma);
a3 = (tau * Kp * ke + Kp * d + C1 * ke + Ai^2 + Ao^2) / (tau * C1 * ma);
a4 = (Kp * ke) / (tau * C1 * ma);
beta = (ksp * Ks * ke * (Ai + Ao)) / (tau * C1 * ma);

% State -Space Matrices

A = [
0,1,0,0;
0,0,1,0;
0,0,0,1;
-a4,-a3,-a2,-a1];

B = [0;0;0;beta];
C = [1,0,0,0];
% State -Space equations
xdot = A * x + B * u;
y = C *x;

== matlab function Q1_part2/Q1-4/MATLAB Function1 ==
  data: xdot output size=4; u input size=1; y output size=1; x input size=4; t input size=1
function [xdot , y] = System_SS_Model(u, x, t)

% Parameter ranges pertaining to the linear transfer function

ke = 75 + 25 * sin(t);
Ks = 0.375 + 0.125 * sin(t);
Kp = 2.5*10^( -12) + 2.5*10^( -12) * sin(t);
C1 = 2*10^( -11) + 1*10^( -11) * sin(t);
d = 700 + 100 * sin(t);
ma = 20.0 + 0.1 * sin(t);
Ai = 0.00203 + 0.0001 * sin(t);
Ao = 0.00152 + 0.00008 * sin(t);
ksp = 0.0012 + 0.0001 * sin(t);
tau = 35 + 5 * sin(t);

% Definig the parameters calculated for the state - space equations
a1 = (tau * (Kp * ma + C1 * d) + (C1 * ma)) / (tau *C1 * ma);
a2 = (tau * (Kp * d + C1 * ke + Ai^2 + Ao^2) + (Kp *ma + C1 * d)) / (tau * C1 * ma);
a3 = (tau * Kp * ke + Kp * d + C1 * ke + Ai^2 + Ao^2) / (tau * C1 * ma);
a4 = (Kp * ke) / (tau * C1 * ma);
beta = (ksp * Ks * ke * (Ai + Ao)) / (tau * C1 * ma);

% State -Space Matrices

A = [
0,1,0,0;
0,0,1,0;
0,0,0,1;
-a4,-a3,-a2,-a1];

B = [0;0;0;beta];
C = [1,0,0,0];
% State -Space equations
xdot = A * x + B * u;
y = C *x;

== matlab function Q1_part2/Q1-5/MATLAB Function1 ==
  data: xdot output size=4; u input size=1; y output size=1; x input size=4; t input size=1
function [xdot , y] = System_SS_Model(u, x, t)

% Parameter ranges pertaining to the linear transfer function

ke = 75 + 25 * sin(t);
Ks = 0.375 + 0.125 * sin(t);
Kp = 2.5*10^( -12) + 2.5*10^( -12) * sin(t);
C1 = 2*10^( -11) + 1*10^( -11) * sin(t);
d = 700 + 100 * sin(t);
ma = 20.0 + 0.1 * sin(t);
Ai = 0.00203 + 0.0001 * sin(t);
Ao = 0.00152 + 0.00008 * sin(t);
ksp = 0.0012 + 0.0001 * sin(t);
tau = 35 + 5 * sin(t);

% Definig the parameters calculated for the state - space equations
a1 = (tau * (Kp * ma + C1 * d) + (C1 * ma)) / (tau *C1 * ma);
a2 = (tau * (Kp * d + C1 * ke + Ai^2 + Ao^2) + (Kp *ma + C1 * d)) / (tau * C1 * ma);
a3 = (tau * Kp * ke + Kp * d + C1 * ke + Ai^2 + Ao^2) / (tau * C1 * ma);
a4 = (Kp * ke) / (tau * C1 * ma);
beta = (ksp * Ks * ke * (Ai + Ao)) / (tau * C1 * ma);

% State -Space Matrices

A = [
0,1,0,0;
0,0,1,0;
0,0,0,1;
-a4,-a3,-a2,-a1];

B = [0;0;0;beta];
C = [1,0,0,0];
% State -Space equations
xdot = A * x + B * u;
y = C *x;

== matlab function Q1_part2/Q2-2/MATLAB Function Q2openloop ==
  data: x1 input size=1; x2 input size=1; x3 input; x4 input; xdot1 output size=1; u input size=1; xdot2 output size=1; w input; xdot3 output; xdot4 output
function [xdot1, xdot2, xdot3, xdot4] = Q2_System_Model(x1, x2, x3, x4, u, w)

% Parameter Values

m1 = 10000;
m2 = 8000;
k = 500000;
c = 5000;

% State-Equations

xdot1 = x3;
xdot2 = x4;
xdot3 = (1 / m1) * (k * (-x1 + x2) + c * (-x3 + x4) + u + w);
xdot4 = (1 / m2) * (k * (x1 - x2) + c * (x3 - x4));

== matlab function Q1_part2/Q2-1/MATLAB Function Q2openloop ==
  data: x1 input size=1; x2 input size=1; x3 input; x4 input; xdot1 output size=1; u input size=1; xdot2 output size=1; w input; xdot3 output; xdot4 output
function [xdot1, xdot2, xdot3, xdot4] = Q2_System_Model(x1, x2, x3, x4, u, w)

% Parameter Values

m1 = 10000;
m2 = 8000;
k = 500000;
c = 5000;

% State-Equations

xdot1 = x3;
xdot2 = x4;
xdot3 = (1 / m1) * (k * (-x1 + x2) + c * (-x3 + x4) + u + w);
xdot4 = (1 / m2) * (k * (x1 - x2) + c * (x3 - x4));

== matlab function Q1_part2/Q2-3/MATLAB Function Q2openloop ==
  data: x1 input size=1; x2 input size=1; x3 input; x4 input; xdot1 output size=1; u input size=1; xdot2 output size=1; w input; xdot3 output; xdot4 output
function [xdot1, xdot2, xdot3, xdot4] = Q2_System_Model(x1, x2, x3, x4, u, w)

% Parameter Values

m1 = 10000;
m2 = 8000;
k = 500000;
c = 5000;

% State-Equations

xdot1 = x3;
xdot2 = x4;
xdot3 = (1 / m1) * (k * (-x1 + x2) + c * (-x3 + x4) + u + w);
xdot4 = (1 / m2) * (k * (x1 - x2) + c * (x3 - x4));
